simulink model "hinfdm"  (Simulink 5.0)
settings: Solver=ode23  SolverMode=SingleTasking  StartTime=0.0  StopTime=200  MaxStep=0.1  RelTol=1e-3  AbsTol=1e-6
PreLoadFcn:
  | hinfdata
values from neighbouring files (symbols this model uses):
  a = mklti(a,b1,b2,c1,c2,d11,d12,d21,d22,Ts,'tss')    [augss.m]    (also in bilin.m = -xx(1,2); des2ss.m = ue'*a*ve; fitgain.m = ss_; h2data.m = [  -1.0285    0.9853   -0.9413    0.0927)
  b = -xx(1,1)    [bilin.m]    (also in clxbode.m = b(:,iu); des2ss.m = ue'*b; dfreqrc.m = p'*b; h2data.m = [         0)
  c = xx(1,3)    [bilin.m]    (also in des2ss.m = c*ve; dfreqrc.m = c*p; h2data.m = [  -1.7786    1.1390         0   -1.0294]; hinfdata.m = [  -1.7786    1.1390         0   -1.0294])
  d = xx(1,4)    [bilin.m]    (also in clxbode.m = d(:,iu); cschur.m = abs(diag(t)); h2data.m = 0; hinfdata.m = 0)
settings Model: Creator=eyarrow  LastModifiedBy=eyarrow  ExtModeMexFile=ext_comm.c  ExtModeTrigMode=oneshot  ExtModeArmWhenConnect=off  ExternalInput=[]  InitialState=[]  SaveTime=off  SaveOutput=off  LimitDataPoints=off  IntegerOverflowMsg=none  BooleanDataType=off  RTWTemplateMakefile=grt_unix.tmf

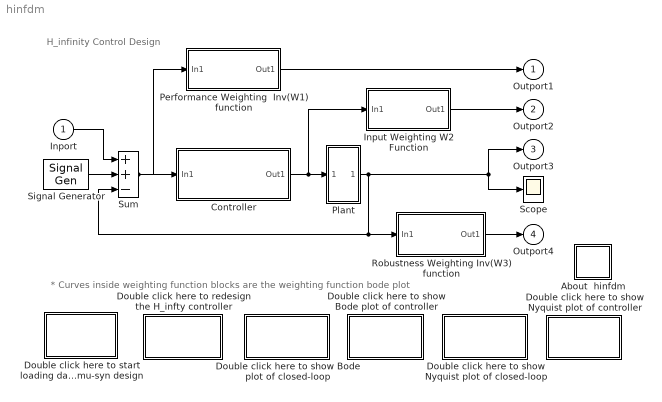
== system hinfdm ==
  note: * Curves inside weighting function blocks are the weighting function bode plot
  note: H_infinity Control Design
  Inport : Inport
  About  hinfdm : Subsystem
      settings: OpenFcn=clc; more(24); help hinfdata; more off
      mask Display: disp('?')
  Controller : Subsystem  mask(H_infty CONTROLLER){@1=ae, @2=be, @3=ce, @4=de}
      mask prompts: @1 "Controller Matrix A:"; @2 "Controller Matrix B:"; @3 "Controller Matrix C:"; @4 "Controller Matrix D:"
      mask help:
      | H_infty controller.
      | (Requires Control Toolbox and RCT)
      mask init:
      | ae=@1; be=@2; ce=@3; de=@4;
      mask Help: H_infty controller design. Mask and unmask this block to see how it works.
      mask Display: disp('H_infty Controller')
  Double click here to redesign the H_infty controller : Subsystem
      settings: OpenFcn=if ~exist('obalreal'),fprintf('\nMust be licensed for RCT Toolbox\n'), else, fprintf('\nCtrl_C to abort RCT Calculation\n\n'); hinfdes1; end
      mask Display: disp('Re-Design')
  Double click here to show Bode plot of closed-loop : Subsystem
      settings: OpenFcn=if ~exist('ae'),fprintf('\nMust Load Data & Design First\n'),else [x,y,z,w]=series(a,b,c,d,ae,be,ce,de);[x,y,z,w]=cloop(x,y,z,w,-1); [x,y,w]=bode(x,y,z,w); clf; subplot(211); loglog(w,x(:,1)); subplot(212); semilogx(w,y(:,1)); subplot(111);end
      mask Display: disp('Closed-Loop\nBode Plot')
  Double click here to show Bode plot of controller : Subsystem
      settings: OpenFcn="if ~exist('ae'),fprintf('\\nMust Load Data & Design First\\n'),else  [x,y,w]=bode(ae,be,ce,de); clf; subplot(211); loglog(w,x); subplot(212); semilogx(w,y); subplot(111); end"
      mask Display: disp('Controller\nBode Plot')
  Double click here to show Nyquist plot of closed-loop : Subsystem
      settings: OpenFcn=if ~exist('ae'), fprintf('\nMust Load Data & Desgin First\n'), else,[x,y,z,w]=feedback(a,b,c,d,ae,be,ce,de,-1); clf, nyquist(x,y,z,w); end
      mask Display: disp('Closed-Loop\nNyquist')
  Double click here to show Nyquist plot of controller : Subsystem
      settings: OpenFcn=if ~exist('ae'), fprintf('\nMust Load Data & Desgin First\n'), else,clf; nyquist(ae,be,ce,de), end
      mask Display: disp('Controller\nNyquist')
  Double click here to start loading data and mu-syn design : Subsystem
      settings: OpenFcn=if ~exist('obalreal'),fprintf('\nMust be licensed for RCT Toolbox\n'), else, fprintf('\nCtrl_C to abort RCT Calculation\n\n'); hinfdata;end
      mask Display: disp('Re-Load\nData')
  Input Weighting W2 Function : Subsystem  mask(polynomial: num/den){@1=num2, @2=den2}
      mask prompts: @1 "numerator:"; @2 "denominator:"
      mask help:
      | Transfer Function
      | numerator and denominator:
      mask init:
      | num2=@1;den2=@2;[ma2,pa2,w2]=bode(num2,den2);
      mask Help: Transfer Function
      mask Display: plot(log10(w2),log10(ma2));
  Performance Weighting  Inv(W1) function : Subsystem  mask(polynomial: num/den){@1=num1, @2=den1}
      mask prompts: @1 "numerator:"; @2 "denominator:"
      mask help:
      | Transfer function
      |  numerator and denominator
      mask init:
      | num1=@1;den1=@2;[ma1,ph1,w1]=bode(num1,den1);
      mask Help: Transfer function
      mask Display: plot(log10(w1),log10(ma1));
  Plant : Subsystem
  Robustness Weighting Inv(W3) function : Subsystem  mask(polynomial: num/den){@1=num3, @2=den3}
      mask prompts: @1 "numerator:"; @2 "denominator:"
      mask help:
      | Transfer Function
      | numerator and denominator:
      mask init:
      | num3=@1;den3=@2;[ma3,ph3,w3]=bode(num3,den3);
      mask Help: Transfer Function
      mask Display: plot(log10(w3),log10(ma3))
  Scope : Scope
      settings: TickLabels=on  TimeRange=10.000000  DataFormat=Array
  Signal Generator : SignalGenerator
  Sum : Sum  Inputs=++-  SaturateOnIntegerOverflow=on  InputSameDT=on
  Outport1 : Outport  InitialOutput=0
  Outport2 : Outport  Port=2  InitialOutput=0
  Outport3 : Outport  Port=3  InitialOutput=0
  Outport4 : Outport  Port=4  InitialOutput=0
  wires:
  Input Weighting W2 Function/1(Out1) -> Outport2/1
  Sum/1 -> Performance Weighting  Inv(W1) function/1(In1), Controller/1(In1)
  Inport/1 -> Sum/1
  Signal Generator/1 -> Sum/2
  Controller/1(Out1) -> Input Weighting W2 Function/1(In1), Plant/1(in)
  Plant/1(out) -> Robustness Weighting Inv(W3) function/1(In1), Sum/3, Scope/1, Outport3/1
  Performance Weighting  Inv(W1) function/1(Out1) -> Outport1/1
  Robustness Weighting Inv(W3) function/1(Out1) -> Outport4/1

== system hinfdm/About  hinfdm ==

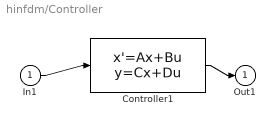
== system hinfdm/Controller ==
  In1 : Inport
  Controller1 : StateSpace  A=ae  B=be  C=ce  D=de
  Out1 : Outport  InitialOutput=0
  wires:
  In1/1 -> Controller1/1
  Controller1/1 -> Out1/1

== system hinfdm/Double click here to redesign the H_infty controller ==

== system hinfdm/Double click here to show Bode plot of closed-loop ==

== system hinfdm/Double click here to show Bode plot of controller ==

== system hinfdm/Double click here to show Nyquist plot of closed-loop ==

== system hinfdm/Double click here to show Nyquist plot of controller ==

== system hinfdm/Double click here to start loading data and mu-syn design ==

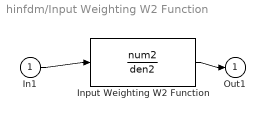
== system hinfdm/Input Weighting W2 Function ==
  In1 : Inport
  Input Weighting W2 Function : TransferFcn  Numerator=num2  Denominator=den2
  Out1 : Outport  InitialOutput=0
  wires:
  In1/1 -> Input Weighting W2 Function/1
  Input Weighting W2 Function/1 -> Out1/1

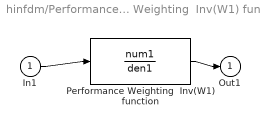
== system hinfdm/Performance Weighting  Inv(W1) function ==
  In1 : Inport
  Performance Weighting  Inv(W1) function : TransferFcn  Numerator=num1  Denominator=den1
  Out1 : Outport  InitialOutput=0
  wires:
  In1/1 -> Performance Weighting  Inv(W1) function/1
  Performance Weighting  Inv(W1) function/1 -> Out1/1

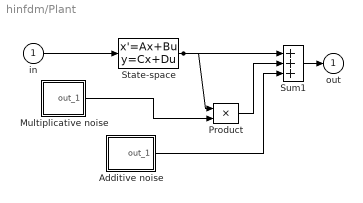
== system hinfdm/Plant ==
  in : Inport
  Additive noise : Subsystem  mask(Input Noise){@1=0.1, @2=1, @3=12345}
      mask prompts: @1 "Noise Variance:"; @2 "Sample Time:"; @3 "Seed"
      mask help:
      | White noise for continuous (s-domain) systems.
      | Band-limited using zero-order-hold.
      mask init:
      | Cov = @1; Ts = @2; seed = @3; r = rand(1,12)-0.5;
      mask Help: Implemented using white noise into Zero Order Hold block. For faster simulation set sample time to highest value possible but in accordance with the fastest dynamics of system.
      mask Display: plot(1:20,rand(1,20))
  Multiplicative noise : Subsystem  mask(Input Noise){@1=0.1, @2=1, @3=6455}
      mask prompts: @1 "Noise Variance:"; @2 "Sample Time:"; @3 "Seed"
      mask help:
      | White noise for continuous (s-domain) systems.
      | Band-limited using zero-order-hold.
      mask init:
      | Cov = @1; Ts = @2; seed = @3; r = rand(1,12)-0.5;
      mask Help: Implemented using white noise into Zero Order Hold block. For faster simulation set sample time to highest value possible but in accordance with the fastest dynamics of system.
      mask Display: plot(1:20,rand(1,20))
  Product : Product  SaturateOnIntegerOverflow=on  InputSameDT=on
  State-space : StateSpace  A=a  B=b  C=c  D=d
  Sum1 : Sum  Inputs=+++  SaturateOnIntegerOverflow=on  InputSameDT=on
  out : Outport  InitialOutput=0
  wires:
  in/1 -> State-space/1
  Sum1/1 -> out/1
  State-space/1 -> Sum1/1, Product/1
  Multiplicative noise/1(out_1) -> Product/2
  Product/1 -> Sum1/2
  Additive noise/1(out_1) -> Sum1/3

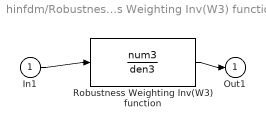
== system hinfdm/Robustness Weighting Inv(W3) function ==
  In1 : Inport
  Robustness Weighting Inv(W3) function : TransferFcn  Numerator=num3  Denominator=den3
  Out1 : Outport  InitialOutput=0
  wires:
  In1/1 -> Robustness Weighting Inv(W3) function/1
  Robustness Weighting Inv(W3) function/1 -> Out1/1

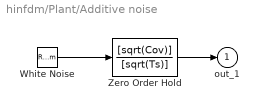
== system hinfdm/Plant/Additive noise ==
  White Noise : RandomNumber  Seed=seed  SampleTime=Ts
  Zero Order Hold : DiscreteTransferFcn  Numerator=[sqrt(Cov)]  Denominator=[sqrt(Ts)]  SampleTime=Ts
  out_1 : Outport  InitialOutput=0
  wires:
  White Noise/1 -> Zero Order Hold/1
  Zero Order Hold/1 -> out_1/1

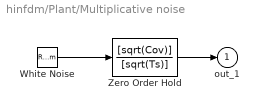
== system hinfdm/Plant/Multiplicative noise ==
  White Noise : RandomNumber  Seed=seed  SampleTime=Ts
  Zero Order Hold : DiscreteTransferFcn  Numerator=[sqrt(Cov)]  Denominator=[sqrt(Ts)]  SampleTime=Ts
  out_1 : Outport  InitialOutput=0
  wires:
  White Noise/1 -> Zero Order Hold/1
  Zero Order Hold/1 -> out_1/1
